simulink model "ECE556Lab1Task3"  (R2013b)
settings: Solver=ode45  StartTime=0.0  StopTime=10.0  RelTol=1e-3
settings Model: Creator=Ben  LastModifiedBy=Ben

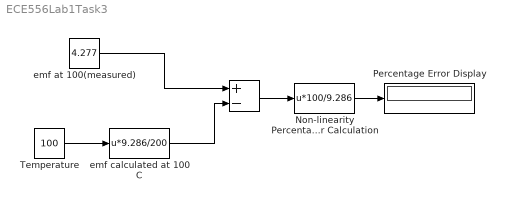
== system ECE556Lab1Task3 ==
  " " : Sum  Inputs=+-
  Non-linearity Percentage Error Calculation : Fcn  Expr=u*100/9.286
  Percentage Error Display : Display
  Temperature : Constant  Value=100
  emf at 100(measured) : Constant  Value=4.277  LockScale=on
  emf calculated at 100 C : Fcn  Expr=u*9.286/200
  wires:
  Temperature/1 -> emf calculated at 100 C/1
  emf calculated at 100 C/1 -> " "/2
  emf at 100(measured)/1 -> " "/1
  " "/1 -> Non-linearity Percentage Error Calculation/1
  Non-linearity Percentage Error Calculation/1 -> Percentage Error Display/1
